simulink model "modeloSimulink"  (R2024b)
settings: Solver=VariableStepAuto  StartTime=0.0  StopTime=5  RelTol=1e-3
settings Model: Creator=Ruben  LastModifiedBy=Ruben
settings DataIOCC: InspectSignalLogs=on  ReturnWorkspaceOutputs=off

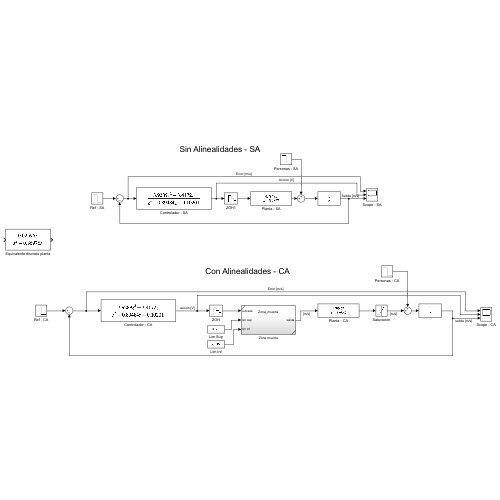
[thumbnail: Simulink's stored preview of the top-level diagram]
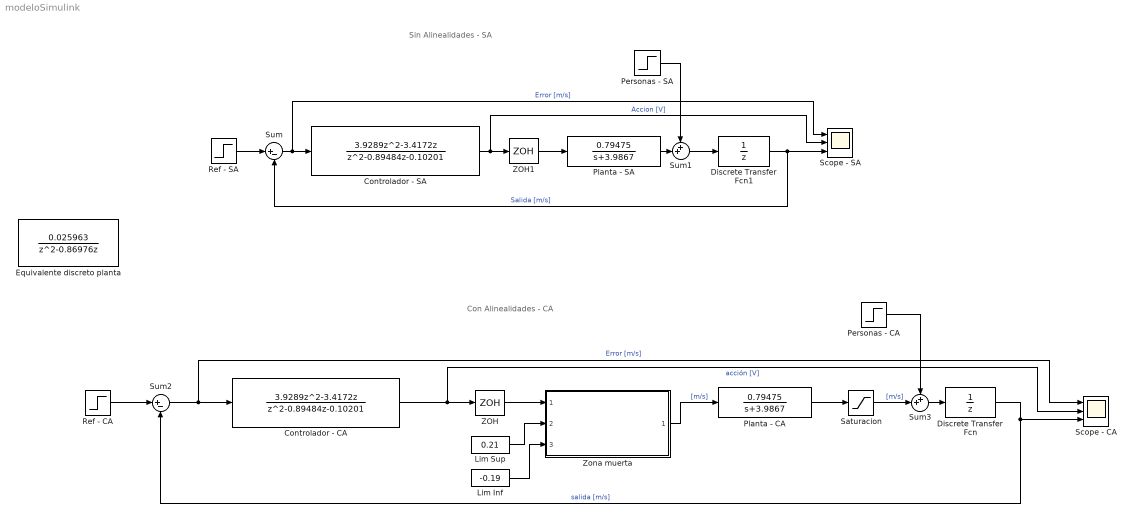
== system modeloSimulink ==
  note: Sin Alinealidades - SA
  note: Con Alinealidades - CA
  Controlador - CA : DiscreteTransferFcn  Numerator=[3.9289 -3.4172 0]  Denominator=[1 -0.89484 -0.10201]
  Controlador - SA : DiscreteTransferFcn  Numerator=[3.9289 -3.4172 0]  Denominator=[1 -0.89484 -0.10201]
  Discrete Transfer Fcn : DiscreteTransferFcn  Denominator=[1 0]
  Discrete Transfer Fcn1 : DiscreteTransferFcn  Denominator=[1 0]
  Equivalente discreto planta : DiscreteTransferFcn  Numerator=[0 0 0.025963]  Denominator=[1 -0.86976 0]
  Lim Inf : Constant  Value=-0.19
  Lim Sup : Constant  Value=0.21
  Personas - CA : Step  Time=2.5  After=-0.2  SampleTime=0.035
  Personas - SA : Step  Time=2.5  After=-0.2  SampleTime=0.035
  Planta - CA : TransferFcn  Numerator=[0 0.79475]  Denominator=[1 3.9867]
  Planta - SA : TransferFcn  Numerator=[0 0.79475]  Denominator=[1 3.9867]
  Ref - CA : Step  Time=0  After=-1  SampleTime=0.035
  Ref - SA : Step  Time=0  After=-1  SampleTime=0.035
  Saturacion : Saturate  UpperLimit=2.11  LowerLimit=-2.11
  Scope - CA : Scope  NumInputPorts=3
  Scope - SA : Scope  NumInputPorts=3
  Sum : Sum  Inputs=|+-
  Sum1 : Sum  Inputs=++|
  Sum2 : Sum  Inputs=|+-
  Sum3 : Sum  Inputs=++|
  ZOH : ZeroOrderHold  SampleTime=-1
  ZOH1 : ZeroOrderHold  SampleTime=-1
  Zona muerta : Subsystem  ReferencedSubsystem=Zona_muerta
  wires:
  Ref - SA/1 -> Sum/1
  Sum/1 -> Scope - SA/1, Controlador - SA/1  "Error [m/s]"
  Sum1/1 -> Discrete Transfer Fcn1/1
  Personas - SA/1 -> Sum1/1
  Ref - CA/1 -> Sum2/1
  Personas - CA/1 -> Sum3/1
  Sum3/1 -> Discrete Transfer Fcn/1
  Discrete Transfer Fcn/1 -> Scope - CA/3, Sum2/2  "salida [m/s]"
  Sum2/1 -> Controlador - CA/1, Scope - CA/1  "Error [m/s]"
  ZOH1/1 -> Planta - SA/1
  Controlador - SA/1 -> Scope - SA/2, ZOH1/1  "Accion [V]"
  Planta - SA/1 -> Sum1/2
  Discrete Transfer Fcn1/1 -> Sum/2, Scope - SA/3  "Salida [m/s]"
  Controlador - CA/1 -> ZOH/1, Scope - CA/2  "acción [V]"
  Lim Inf/1 -> Zona muerta/3
  Lim Sup/1 -> Zona muerta/2
  Zona muerta/1 -> Planta - CA/1  "[m/s]"
  Saturacion/1 -> Sum3/2  "[m/s]"
  ZOH/1 -> Zona muerta/1
  Planta - CA/1 -> Saturacion/1
